simulink model "LAB_3_NO_1_DAVID_AND_ABELLA_BLOCK_DIAGRAM_ALG"  (R2024a)
settings: Solver=VariableStepAuto  StartTime=0.0  StopTime=20.0  RelTol=1e-3
values from neighbouring files (symbols this model uses):
  G1_den = [1 0 0]    [LAB_3_NO_1_DAVID_AND_ABELLA.m]
  G1_num = [0 0 1]    [LAB_3_NO_1_DAVID_AND_ABELLA.m]
  G2_den = [1 1]    [LAB_3_NO_1_DAVID_AND_ABELLA.m]
  G2_den_sum = conv(G2_den, G2_num)    [LAB_3_NO_1_DAVID_AND_ABELLA.m]
  G2_num = [0 1]    [LAB_3_NO_1_DAVID_AND_ABELLA.m]
  G2_num_sum = conv(G2_num, G2_den)    [LAB_3_NO_1_DAVID_AND_ABELLA.m]
  G3_den = [1 0]    [LAB_3_NO_1_DAVID_AND_ABELLA.m]
  G3_num = [0 1]    [LAB_3_NO_1_DAVID_AND_ABELLA.m]
  GH2_den = conv(G2_den, H2_den)    [LAB_3_NO_1_DAVID_AND_ABELLA.m]
  GH2_num = conv(G2_num, H2_num)    [LAB_3_NO_1_DAVID_AND_ABELLA.m]
  H1_den = [1 0]    [LAB_3_NO_1_DAVID_AND_ABELLA.m]
  H1_num = [0 1]    [LAB_3_NO_1_DAVID_AND_ABELLA.m]
  H2_den = [1 -1]    [LAB_3_NO_1_DAVID_AND_ABELLA.m]
  H2_num = [0 1]    [LAB_3_NO_1_DAVID_AND_ABELLA.m]
  H3_den = [1 -2]    [LAB_3_NO_1_DAVID_AND_ABELLA.m]
  H3_num = [0 1]    [LAB_3_NO_1_DAVID_AND_ABELLA.m]
  TF1_den = conv(G1_den, TF2_den)    [LAB_3_NO_1_DAVID_AND_ABELLA.m]
  TF1_num = conv(G1_num, TF2_num)    [LAB_3_NO_1_DAVID_AND_ABELLA.m]
  TF3_den = conv(G3_den, TF3_add)    [LAB_3_NO_1_DAVID_AND_ABELLA.m]
  TF3_num = conv(GH3_den, GH3_num)    [LAB_3_NO_1_DAVID_AND_ABELLA.m]
  TF4_den = conv(TF3_den, G2_den_sum)    [LAB_3_NO_1_DAVID_AND_ABELLA.m]
  TF4_num = conv(TF3_num, G2_num_sum)    [LAB_3_NO_1_DAVID_AND_ABELLA.m]
  TF5_den = conv(TF1_den, TF5_add)    [LAB_3_NO_1_DAVID_AND_ABELLA.m]
  TF5_num = conv(TF1_num, TFH1_den)    [LAB_3_NO_1_DAVID_AND_ABELLA.m]
  TF_den = conv(TF5_den, TF4_den)    [LAB_3_NO_1_DAVID_AND_ABELLA.m]    (also in Lab_3_No_2_ENRIQUEZ_JK_and_NAVARRO_AE.m = conv(TF_n_2,TF_d_1))
  TF_num = conv(TF5_num, TF4_num)    [LAB_3_NO_1_DAVID_AND_ABELLA.m]    (also in Lab_3_No_2_ENRIQUEZ_JK_and_NAVARRO_AE.m = conv(TF_n_1,TF_d_2))
settings Model: Creator=PC  LastModifiedBy=PC

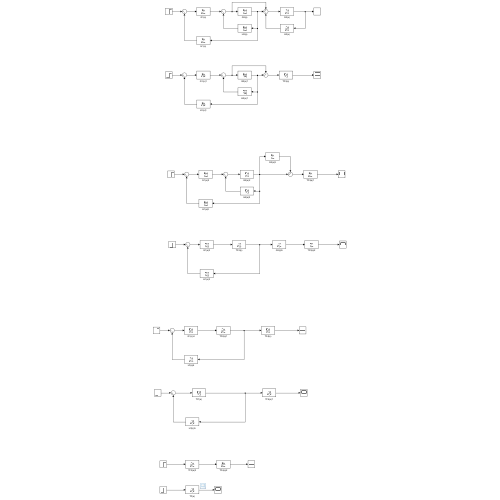
[thumbnail: Simulink's stored preview of the top-level diagram]
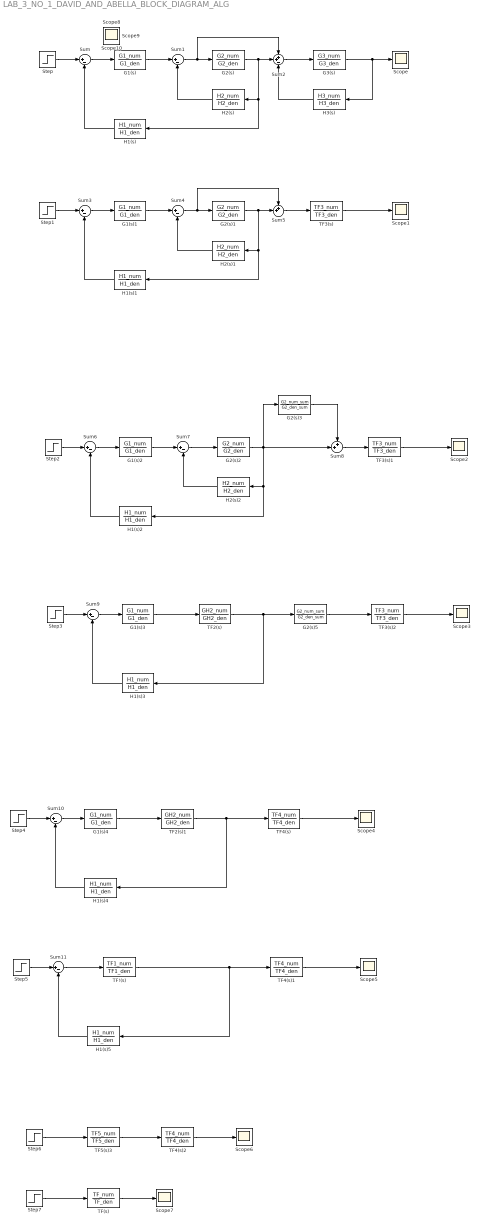
== system LAB_3_NO_1_DAVID_AND_ABELLA_BLOCK_DIAGRAM_ALG ==
  G1(s){,1..4} (5 alike) : TransferFcn  Numerator=G1_num  Denominator=G1_den
  G2(s) : TransferFcn  Numerator=G2_num  Denominator=G2_den
  G2(s)1 : TransferFcn  Numerator=G2_num  Denominator=G2_den
  G2(s)2 : TransferFcn  Numerator=G2_num  Denominator=G2_den
  G2(s)3 : TransferFcn  Numerator=G2_num_sum  Denominator=G2_den_sum
  G2(s)5 : TransferFcn  Numerator=G2_num_sum  Denominator=G2_den_sum
  G3(s) : TransferFcn  Numerator=G3_num  Denominator=G3_den
  H1(s){,1..5} (6 alike) : TransferFcn  Numerator=H1_num  Denominator=H1_den
  H2(s) : TransferFcn  Numerator=H2_num  Denominator=H2_den
  H2(s)1 : TransferFcn  Numerator=H2_num  Denominator=H2_den
  H2(s)2 : TransferFcn  Numerator=H2_num  Denominator=H2_den
  H3(s) : TransferFcn  Numerator=H3_num  Denominator=H3_den
  Scope{,1..10} (11 alike) : Scope
  Step{,1..6} (7 alike) : Step  SampleTime=0
  Step7 : Step  Time=0  Before=0.1  SampleTime=0
  Sum{,1,3..4,6..7,9..11} (9 alike) : Sum  Inputs=|+-
  Sum2 : Sum  Inputs=++-
  Sum5 : Sum  Inputs=++|
  Sum8 : Sum  Inputs=++|
  TF!(s) : TransferFcn  Numerator=TF1_num  Denominator=TF1_den
  TF(s) : TransferFcn  Numerator=TF_num  Denominator=TF_den
  TF2(s) : TransferFcn  Numerator=GH2_num  Denominator=GH2_den
  TF2(s)1 : TransferFcn  Numerator=GH2_num  Denominator=GH2_den
  TF3(s) : TransferFcn  Numerator=TF3_num  Denominator=TF3_den
  TF3(s)1 : TransferFcn  Numerator=TF3_num  Denominator=TF3_den
  TF3(s)2 : TransferFcn  Numerator=TF3_num  Denominator=TF3_den
  TF4(s) : TransferFcn  Numerator=TF4_num  Denominator=TF4_den
  TF4(s)1 : TransferFcn  Numerator=TF4_num  Denominator=TF4_den
  TF4(s)2 : TransferFcn  Numerator=TF4_num  Denominator=TF4_den
  TF5(s)3 : TransferFcn  Numerator=TF5_num  Denominator=TF5_den
  wires:
  G3(s)/1 -> H3(s)/1, Scope/1
  Step/1 -> Sum/1
  Sum/1 -> G1(s)/1
  G1(s)/1 -> Sum1/1
  Sum1/1 -> Sum2/1, G2(s)/1
  G2(s)/1 -> H1(s)/1, H2(s)/1, Sum2/2
  Sum2/1 -> G3(s)/1
  H3(s)/1 -> Sum2/3
  H2(s)/1 -> Sum1/2
  H1(s)/1 -> Sum/2
  Sum3/1 -> G1(s)1/1
  G2(s)1/1 -> Sum5/2, H1(s)1/1, H2(s)1/1
  H1(s)1/1 -> Sum3/2
  H2(s)1/1 -> Sum4/2
  Sum4/1 -> Sum5/1, G2(s)1/1
  Step1/1 -> Sum3/1
  G1(s)1/1 -> Sum4/1
  Sum5/1 -> TF3(s)/1
  TF3(s)/1 -> Scope1/1
  Sum8/1 -> TF3(s)1/1
  Sum6/1 -> G1(s)2/1
  G1(s)2/1 -> Sum7/1
  Step2/1 -> Sum6/1
  Sum7/1 -> G2(s)2/1
  H1(s)2/1 -> Sum6/2
  G2(s)2/1 -> G2(s)3/1, Sum8/2, H1(s)2/1, H2(s)2/1
  H2(s)2/1 -> Sum7/2
  TF3(s)1/1 -> Scope2/1
  G2(s)3/1 -> Sum8/1
  TF3(s)2/1 -> Scope3/1
  Sum9/1 -> G1(s)3/1
  H1(s)3/1 -> Sum9/2
  Step3/1 -> Sum9/1
  G2(s)5/1 -> TF3(s)2/1
  TF2(s)/1 -> H1(s)3/1, G2(s)5/1
  G1(s)3/1 -> TF2(s)/1
  H1(s)4/1 -> Sum10/2
  Step4/1 -> Sum10/1
  G1(s)4/1 -> TF2(s)1/1
  Sum10/1 -> G1(s)4/1
  TF2(s)1/1 -> TF4(s)/1, H1(s)4/1
  TF4(s)/1 -> Scope4/1
  TF4(s)1/1 -> Scope5/1
  TF!(s)/1 -> TF4(s)1/1, H1(s)5/1
  H1(s)5/1 -> Sum11/2
  Sum11/1 -> TF!(s)/1
  Step5/1 -> Sum11/1
  TF4(s)2/1 -> Scope6/1
  Step6/1 -> TF5(s)3/1
  TF5(s)3/1 -> TF4(s)2/1
  Step7/1 -> TF(s)/1
  TF(s)/1 -> Scope7/1
